simulink model "MyS_Tarea1"  (R2024a)
settings: Solver=VariableStepAuto  StartTime=0.0  StopTime=10  MaxStep=0.0001  RelTol=1e-3
InitFcn:
  | m1=0.2;
  | l1=0.3;
  | m2=0.1;
  | l2=0.25;
  | g=9.81;

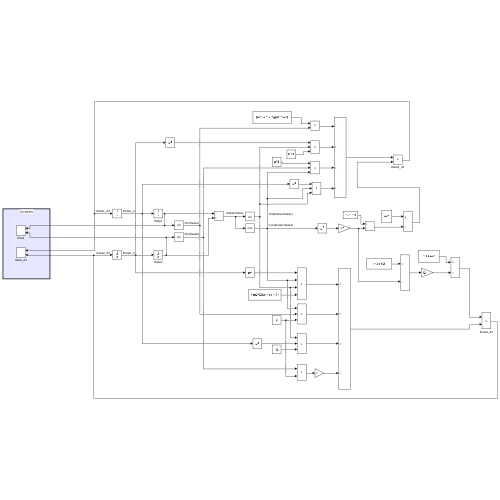
[thumbnail: Simulink's stored preview of the top-level diagram]
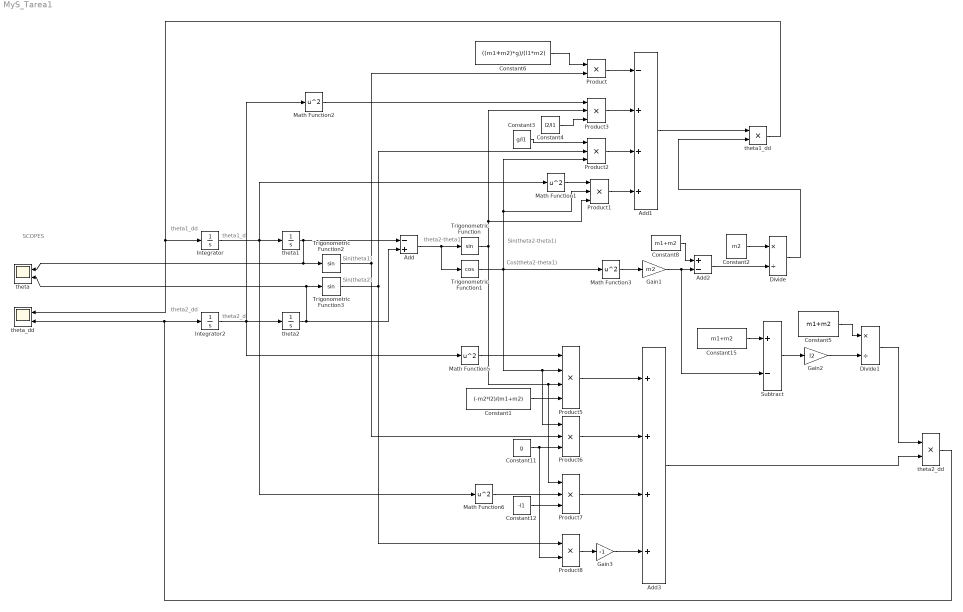
== system MyS_Tarea1 ==
  note: SCOPES
  note: Cos(theta2-theta1)
  note: Sin(theta2-theta1)
  note: Sin(theta1)
  note: theta2-theta1
  note: theta1_dd
  note: theta1_d
  note: theta2_dd
  note: theta2_d
  note: Sin(theta2)
  Add : Sum  Inputs=-+
  Add1 : Sum  Inputs=-+++
  Add2 : Sum  Inputs=+-
  Add3 : Sum  Inputs=++++
  Constant1 : Constant  Value=(-m2*l2)/(m1+m2)
  Constant11 : Constant  Value=g
  Constant12 : Constant  Value=-l1
  Constant15 : Constant  Value=m1+m2
  Constant2 : Constant  Value=m2
  Constant3 : Constant  Value=g/l1
  Constant4 : Constant  Value=l2/l1
  Constant5 : Constant  Value=m1+m2
  Constant6 : Constant  Value=((m1+m2)*g)/(l1*m2)
  Constant8 : Constant  Value=m1+m2
  Divide : Product  Inputs=*/
  Divide1 : Product  Inputs=*/
  Gain1 : Gain  Gain=m2
  Gain2 : Gain  Gain=l2
  Gain3 : Gain  Gain=-1
  Integrator : Integrator
  Integrator2 : Integrator
  Math Function{1..3,5..6} (5 alike) : Math  Operator=square
  Product : Product
  Product{1..3,6..7} (5 alike) : Product  Inputs=3
  Product5 : Product  Inputs=4
  Product8 : Product
  Subtract : Sum  Inputs=+-
  Trigonometric Function : Trigonometry
  Trigonometric Function1 : Trigonometry  Operator=cos
  Trigonometric Function2 : Trigonometry
  Trigonometric Function3 : Trigonometry
  theta : Scope  NumInputPorts=2
  theta1 : Integrator
  theta1_dd : Product
  theta2 : Integrator  InitialCondition=(35*pi)/180
  theta2_dd : Product
  theta_dd : Scope  NumInputPorts=2
  wires:
  theta1/1 -> theta/1, Trigonometric Function2/1, Add/1
  theta2/1 -> theta/2, Trigonometric Function3/1, Add/2
  Add/1 -> Trigonometric Function/1, Trigonometric Function1/1
  Trigonometric Function1/1 -> Product6/1, Product5/2, Math Function3/1, Product2/3, Product1/2
  Math Function1/1 -> Product1/1
  Constant3/1 -> Product2/1
  Trigonometric Function3/1 -> Product8/1, Product2/2
  Trigonometric Function/1 -> Product7/1, Product5/3, Product3/2, Product1/3
  Constant4/1 -> Product3/3
  Math Function2/1 -> Product3/1
  Constant6/1 -> Product/1
  Trigonometric Function2/1 -> Product/2, Product6/2
  Product/1 -> Add1/1
  Product3/1 -> Add1/2
  Product2/1 -> Add1/3
  Product1/1 -> Add1/4
  Math Function3/1 -> Gain1/1
  Constant8/1 -> Add2/1
  Add1/1 -> theta1_dd/1
  theta1_dd/1 -> Integrator/1, theta_dd/1
  Math Function5/1 -> Product5/1
  Integrator2/1 -> theta2/1, Math Function5/1, Math Function2/1
  Constant11/1 -> Product8/2, Product6/3
  Constant12/1 -> Product7/3
  Constant1/1 -> Product5/4
  Integrator/1 -> theta1/1, Math Function1/1, Math Function6/1
  Math Function6/1 -> Product7/2
  Product8/1 -> Gain3/1
  Product5/1 -> Add3/1
  Gain3/1 -> Add3/4
  Product7/1 -> Add3/3
  Product6/1 -> Add3/2
  Constant15/1 -> Subtract/1
  Gain1/1 -> Subtract/2, Add2/2
  Divide1/1 -> theta2_dd/1
  Add3/1 -> theta2_dd/2
  theta2_dd/1 -> theta_dd/2, Integrator2/1
  Constant2/1 -> Divide/1
  Add2/1 -> Divide/2
  Divide/1 -> theta1_dd/2
  Subtract/1 -> Gain2/1
  Gain2/1 -> Divide1/2
  Constant5/1 -> Divide1/1
